simulink subsystem "magSensor2CM"  (R2021a)
settings: Solver=VariableStepAuto  StartTime=0.0  StopTime=10.0  RelTol=1e-3
libraries: attitude_library x2
settings Model: Creator=Laura  LastModifiedBy=Laura

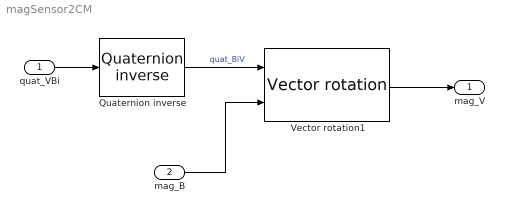
== system magSensor2CM ==
  quat_VBi : Inport
  mag_B : Inport  Port=2
  Quaternion inverse : attitude_library/Quaternion inverse  SystemSampleTime=-1  VariantActivationTime=update diagram  Latency=0  AutoFrameSizeCalculation=off
      settings: SourceProductName=Attitude library
  Vector rotation1 : attitude_library/Vector rotation  SystemSampleTime=-1  VariantActivationTime=update diagram  Latency=0  AutoFrameSizeCalculation=off
      settings: SourceProductName=Attitude library
  mag_V : Outport
  wires:
  Quaternion inverse/1 -> Vector rotation1/1  "quat_BiV"
  mag_B/1 -> Vector rotation1/2
  Vector rotation1/1 -> mag_V/1
  quat_VBi/1 -> Quaternion inverse/1
